simulink model "Integral_Controller"  (R2022a)
settings: Solver=VariableStepAuto  StartTime=0.0  StopTime=30  RelTol=1e-3
values from neighbouring files (symbols this model uses):
  A = [0 0 1 0 0 ... (first row only)    [DesignProjectP2.m]    (also in DesignProjectP3.m; DesignProject_OffsetP3.m; mpc_example_regulation.m = [ 	 0,       0,              1,  0, 0; 	 0,       0,        ; mpc_example_tracking.m = [ 	 0,       0,              1,  0, 0; 	 0,       0,        )
  A_aug = [zeros(1, 1) [0 1 0 0 0] ... (first row only)    [DesignProjectP2.m]    (also in DesignProjectP3.m; DesignProject_OffsetP3.m; mpc_example_regulation.m; phase2_emc.m)
  B = [0;0;0;0;1/La]    [DesignProjectP2.m]    (also in DesignProjectP3.m; DesignProject_OffsetP3.m; mpc_example_regulation.m = [0; 0; 0; 0; 1/La]; mpc_example_tracking.m = [0; 0; 0; 0; 1/La])
  B_aug = [zeros(1,1); B]    [DesignProjectP2.m]    (also in DesignProjectP3.m; DesignProject_OffsetP3.m; mpc_example_regulation.m; phase2_emc.m)
  init = [theta_m_init; theta_l_init; thetadot_m_init; thetadot_l_init; Ia_init]    [ELEN90064_Project_Parameters.m]
  K = K(2:6)    [DesignProjectP2.m]    (also in DesignProjectP3.m; DesignProject_OffsetP3.m = K_dist(2:6); phase2_emc.m = place(A,B,desired_poles))
  Ki = K(1)    [DesignProjectP2.m]    (also in DesignProjectP3.m; DesignProject_OffsetP3.m = K_dist(1))
settings Model: Creator=yang  LastModifiedBy=Admin

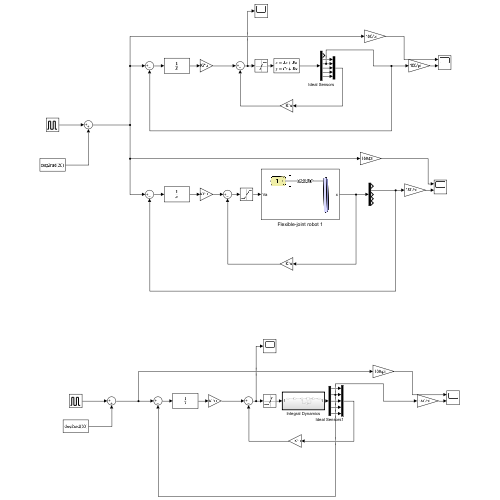
[thumbnail: Simulink's stored preview of the top-level diagram]
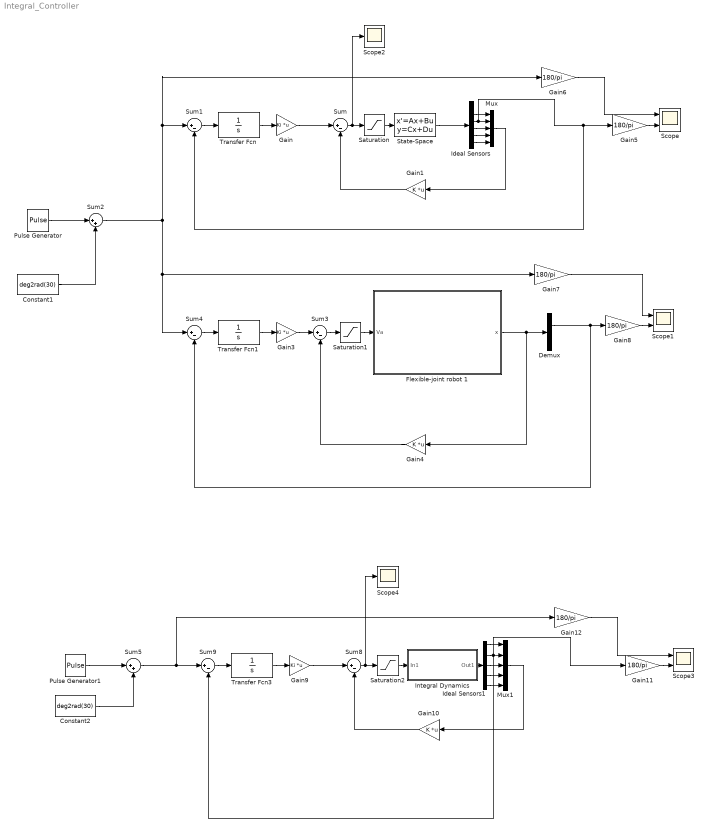
== system Integral_Controller ==
  Constant1 : Constant  Value=deg2rad(30)
  Constant2 : Constant  Value=deg2rad(30)
  Demux : Demux  Outputs=5
  Flexible-joint robot 1 : Subsystem
      mask Display: image('$imagefile'); % Use "Edit Image" on toolstrip to change.
  Gain : Gain  Gain=Ki  Multiplication=Matrix(K*u)
  Gain1 : Gain  Gain=K  Multiplication=Matrix(K*u)
  Gain10 : Gain  Gain=K  Multiplication=Matrix(K*u)
  Gain{5..8,11..12} (6 alike) : Gain  Gain=180/pi
  Gain3 : Gain  Gain=Ki  Multiplication=Matrix(K*u)
  Gain4 : Gain  Gain=K  Multiplication=Matrix(K*u)
  Gain9 : Gain  Gain=Ki  Multiplication=Matrix(K*u)
  Ideal Sensors : Demux  Outputs=6
  Ideal Sensors1 : Demux  Outputs=5
  Integral Dynamics : Subsystem  TreatAsAtomicUnit=on
  Mux : Mux  Inputs=5
  Mux1 : Mux  Inputs=5
  Pulse Generator : DiscretePulseGenerator  PulseType=Time based  Amplitude=deg2rad(30)  Period=10  PulseWidth=50
  Pulse Generator1 : DiscretePulseGenerator  PulseType=Time based  Amplitude=deg2rad(30)  Period=10  PulseWidth=50
  Saturation : Saturate  UpperLimit=6  LowerLimit=-6
  Saturation1 : Saturate  UpperLimit=6  LowerLimit=-6
  Saturation2 : Saturate  UpperLimit=6  LowerLimit=-6
  Scope : Scope  NumInputPorts=2
  Scope1 : Scope  NumInputPorts=2
  Scope2 : Scope
  Scope3 : Scope  NumInputPorts=2
  Scope4 : Scope
  State-Space : StateSpace  A=A_aug  B=B_aug  C=eye(6)  D=zeros(6,1)  InitialCondition=0
  Sum{,1,3..4,8..9} (6 alike) : Sum  Inputs=|+-
  Sum2 : Sum  Inputs=|++
  Sum5 : Sum  Inputs=|++
  Transfer Fcn : TransferFcn  Denominator=[1 0]
  Transfer Fcn1 : TransferFcn  Denominator=[1 0]
  Transfer Fcn3 : TransferFcn  Denominator=[1 0]
  wires:
  Transfer Fcn/1 -> Gain/1
  Gain1/1 -> Sum/2
  Sum1/1 -> Transfer Fcn/1
  State-Space/1 -> Ideal Sensors/1
  Ideal Sensors/2 -> Mux/1
  Ideal Sensors/4 -> Mux/3
  Ideal Sensors/5 -> Mux/4
  Ideal Sensors/6 -> Mux/5
  Mux/1 -> Gain1/1
  Ideal Sensors/3 -> Sum1/2, Gain5/1, Mux/2
  Pulse Generator/1 -> Sum2/1
  Constant1/1 -> Sum2/2
  Sum2/1 -> Sum4/1, Gain7/1, Gain6/1, Sum1/1
  Demux/2 -> Sum4/2, Gain8/1
  Gain4/1 -> Sum3/2
  Sum4/1 -> Transfer Fcn1/1
  Transfer Fcn1/1 -> Gain3/1
  Gain3/1 -> Sum3/1
  Flexible-joint robot 1/1(x) -> Demux/1, Gain4/1
  Gain/1 -> Sum/1
  Sum/1 -> Scope2/1, Saturation/1
  Saturation/1 -> State-Space/1
  Sum3/1 -> Saturation1/1
  Saturation1/1 -> Flexible-joint robot 1/1(Va)
  Gain5/1 -> Scope/2
  Gain6/1 -> Scope/1
  Gain7/1 -> Scope1/1
  Gain8/1 -> Scope1/2
  Constant2/1 -> Sum5/2
  Pulse Generator1/1 -> Sum5/1
  Sum9/1 -> Transfer Fcn3/1
  Transfer Fcn3/1 -> Gain9/1
  Gain10/1 -> Sum8/2
  Sum8/1 -> Scope4/1, Saturation2/1
  Saturation2/1 -> Integral Dynamics/1(In1)
  Gain9/1 -> Sum8/1
  Sum5/1 -> Gain12/1, Sum9/1
  Gain11/1 -> Scope3/2
  Integral Dynamics/1(Out1) -> Ideal Sensors1/1
  Gain12/1 -> Scope3/1
  Mux1/1 -> Gain10/1
  Ideal Sensors1/1 -> Mux1/1
  Ideal Sensors1/2 -> Gain11/1, Sum9/2, Mux1/2
  Ideal Sensors1/3 -> Mux1/3
  Ideal Sensors1/4 -> Mux1/4
  Ideal Sensors1/5 -> Mux1/5

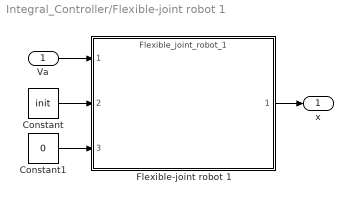
== system Integral_Controller/Flexible-joint robot 1 ==
  Va : Inport
  Constant : Constant  Value=init
  Constant1 : Constant  Value=0
  Flexible-joint robot 1 : ModelReference  ModelNameDialog=Flexible_joint_robot_1  ModelReferenceVersion=1.65  CopyOfModelProtected=on
  x : Outport
  wires:
  Constant/1 -> Flexible-joint robot 1/2
  Constant1/1 -> Flexible-joint robot 1/3
  Flexible-joint robot 1/1 -> x/1
  Va/1 -> Flexible-joint robot 1/1

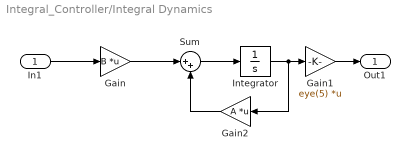
== system Integral_Controller/Integral Dynamics ==
  In1 : Inport
  Gain : Gain  Gain=B  Multiplication=Matrix(K*u)
  Gain1 : Gain  Gain=eye(5)  Multiplication=Matrix(K*u)
  Gain2 : Gain  Gain=A  Multiplication=Matrix(K*u)
  Integrator : Integrator
  Sum : Sum  Inputs=|++
  Out1 : Outport
  wires:
  In1/1 -> Gain/1
  Gain/1 -> Sum/1
  Sum/1 -> Integrator/1
  Integrator/1 -> Gain2/1, Gain1/1
  Gain1/1 -> Out1/1
  Gain2/1 -> Sum/2
